simulink model "lab2"  (R2018b)
settings: Solver=ode4  StartTime=0.0  StopTime=10.0  FixedStep=2^-7  RelTol=1e-3
libraries: simulink x2
settings Model: Creator=vandavv  LastModifiedBy=vandavv

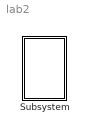
== system lab2 ==
  Subsystem : Subsystem  mask{x0=0, y0=5, vx=10, vy=0, M=100, G=9.81, R=2, RS=0.2}

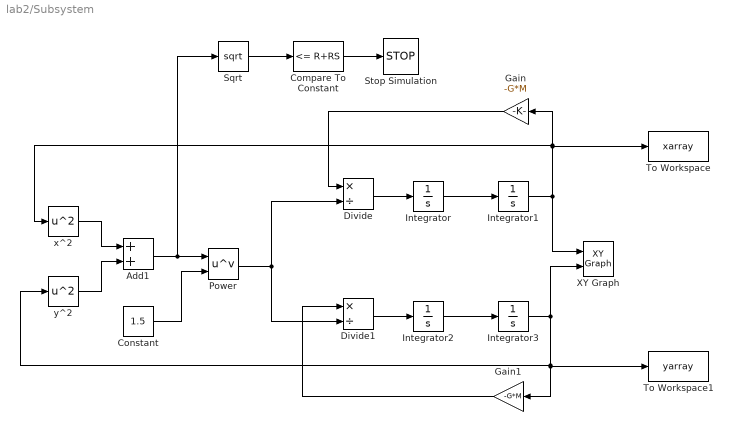
== system lab2/Subsystem ==
  Add1 : Sum
  Compare To Constant : simulink/Logic and Bit Operations/Compare To Constant  relop=<=  const=R+RS  OutDataTypeStr=boolean
  Constant : Constant  Value=1.5
  Divide : Product  Inputs=*/
  Divide1 : Product  Inputs=*/
  Gain : Gain  Gain=-G*M
  Gain1 : Gain  Gain=-G*M
  Integrator : Integrator  InitialCondition=vx
  Integrator1 : Integrator  InitialCondition=x0
  Integrator2 : Integrator  InitialCondition=vy
  Integrator3 : Integrator  InitialCondition=y0
  Power : Math  Operator=pow  SaturateOnIntegerOverflow=on
  Sqrt : Sqrt  SaturateOnIntegerOverflow=on
  Stop Simulation : Stop
  To Workspace : ToWorkspace  VariableName=xarray  SampleTime=-1
  To Workspace1 : ToWorkspace  VariableName=yarray  SampleTime=-1
  XY Graph : simulink/Sinks/XY Graph  xmin=-10  xmax=10  ymin=-10  ymax=10  st=-1
  x^2 : Math  Operator=square  RndMeth=Zero  SaturateOnIntegerOverflow=on
  y^2 : Math  Operator=square  RndMeth=Zero  SaturateOnIntegerOverflow=on
  wires:
  Integrator2/1 -> Integrator3/1
  Divide1/1 -> Integrator2/1
  Integrator/1 -> Integrator1/1
  Divide/1 -> Integrator/1
  Integrator3/1 -> Gain1/1, To Workspace1/1, y^2/1, XY Graph/2
  Gain1/1 -> Divide1/1
  x^2/1 -> Add1/1
  Power/1 -> Divide/2, Divide1/2
  Gain/1 -> Divide/1
  Add1/1 -> Sqrt/1, Power/1
  y^2/1 -> Add1/2
  Integrator1/1 -> XY Graph/1, Gain/1, x^2/1, To Workspace/1
  Constant/1 -> Power/2
  Sqrt/1 -> Compare To Constant/1
  Compare To Constant/1 -> Stop Simulation/1
